simulink model "Failure_management_system"  (R2022b)
settings: Solver=VariableStepAuto  StartTime=0.0  StopTime=100  RelTol=1e-3
model workspace (MAT data in the model file):
  SnqAcq_FailMaxC_C = 2
  SnqAcq_WarnMaxC_C = 150
  SnrAcq_FailCDec_C = 0.2
  SnrAcq_FailCInc_C = 0.2
  SnrAcq_WarnCDec_C = 0.01
  SnrAcq_WarnCInc_C = 0.01
  SnrAcq_sdlDgo_DiagSrv_C = 0.1
  SnrAcq_sdlLow_SnrRead_C = 0.02
  SnrAcq_vMaxClampHys_C = 0.14
  SnrAcq_vMaxClamp_C = 14
  SnrAcq_vMaxLim_C = 16
  SnrAcq_vMinClampHys_C = 0.1
  SnrAcq_vMinClamp_C = 10
  SnrAcq_vMinLim_C = 6
undefined symbols (not defined in the file): sigbuilder_block
libraries: simulink x3
settings Model: NumberOfSteps=20  Creator=Mohamed Wahdan  LastModifiedBy=Mohamed Wahdan

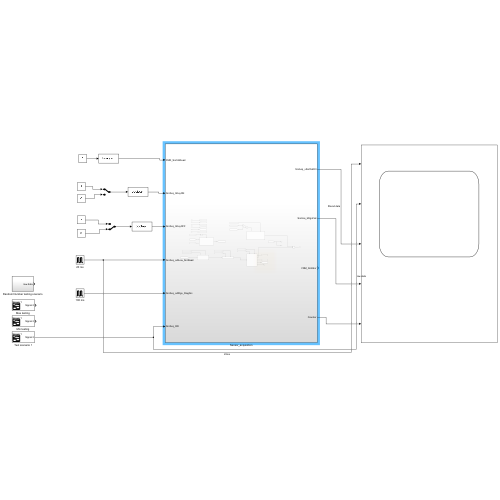
[thumbnail: Simulink's stored preview of the top-level diagram]
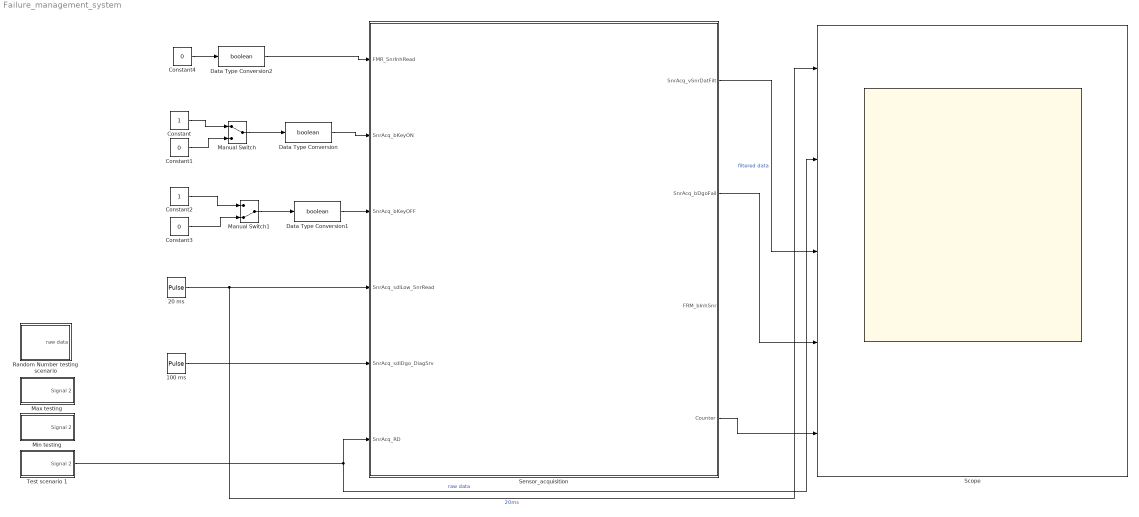
== system Failure_management_system ==
  100 ms : DiscretePulseGenerator  PulseType=Time based  Period=0.1  PulseWidth=50  SampleTime=SnrAcq_sdlDgo_DiagSrv_C
  20 ms : DiscretePulseGenerator  PulseType=Time based  Period=0.02  PulseWidth=50  SampleTime=SnrAcq_sdlLow_SnrRead_C
  Constant : Constant
  Constant1 : Constant  Value=0
  Constant2 : Constant
  Constant3 : Constant  Value=0
  Constant4 : Constant  Value=0
  Data Type Conversion : DataTypeConversion  OutDataTypeStr=boolean  SaturateOnIntegerOverflow=off  RndMeth=Floor
  Data Type Conversion1 : DataTypeConversion  OutDataTypeStr=boolean  SaturateOnIntegerOverflow=off  RndMeth=Floor
  Data Type Conversion2 : DataTypeConversion  OutDataTypeStr=boolean  SaturateOnIntegerOverflow=off  RndMeth=Floor
  Manual Switch : ManualSwitch
  Manual Switch1 : ManualSwitch  CurrentSetting=0
  "Max testing " : Subsystem  Tag=STV Subsys  LoadFcn=sigbuilder_block('load');  StartFcn=sigbuilder_block('start');  StopFcn=sigbuilder_block('stop');  ClipboardFcn=sigbuilder_block('clipboard');  mask(Sigbuilder block){tuvar=[0:10]}
      mask help: Simulink:masks:SigbuilderBlock_MD
      mask init:
      | if ~strcmp(get_param(bdroot(gcbh),'SimulationStatus'),'stopped') tuvar = sigbuilder_block('maskInit'); end
      settings: CopyFcn=sigbuilder_block('copy');  DeleteFcn=sigbuilder_block('delete');  ModelCloseFcn=sigbuilder_block('modelClose');  PreSaveFcn=sigbuilder_block('preSave');  PauseFcn=sigbuilder_block('pause');  ContinueFcn=sigbuilder_block('continue');  NameChangeFcn=sigbuilder_block('namechange');  OpenFcn=sigbuilder_block('open',[6 36 1428 675.75 ]);  CloseFcn=sigbuilder_block('close');
      mask Display: plot(0, 0, 100, 100,[2, 2, 32, 32, 2], [68, 8, 8, 68, 68],[32, 2], [38, 38], [32, 19, 2],[53, 60, 44], [32, 17, 17, 2],[16, 16, 31, 31]);txt = getActiveGroup(gcbh);text(2, 100, txt,'verticalAlignment', 'top');
  "Min testing " : Subsystem  Tag=STV Subsys  LoadFcn=sigbuilder_block('load');  StartFcn=sigbuilder_block('start');  StopFcn=sigbuilder_block('stop');  ClipboardFcn=sigbuilder_block('clipboard');  mask(Sigbuilder block){tuvar=[0:10]}
      mask help: Simulink:masks:SigbuilderBlock_MD
      mask init:
      | if ~strcmp(get_param(bdroot(gcbh),'SimulationStatus'),'stopped') tuvar = sigbuilder_block('maskInit'); end
      settings: CopyFcn=sigbuilder_block('copy');  DeleteFcn=sigbuilder_block('delete');  ModelCloseFcn=sigbuilder_block('modelClose');  PreSaveFcn=sigbuilder_block('preSave');  PauseFcn=sigbuilder_block('pause');  ContinueFcn=sigbuilder_block('continue');  NameChangeFcn=sigbuilder_block('namechange');  OpenFcn=sigbuilder_block('open',[6 36 1428 675.75 ]);  CloseFcn=sigbuilder_block('close');
      mask Display: plot(0, 0, 100, 100,[2, 2, 32, 32, 2], [68, 8, 8, 68, 68],[32, 2], [38, 38], [32, 19, 2],[53, 60, 44], [32, 17, 17, 2],[16, 16, 31, 31]);txt = getActiveGroup(gcbh);text(2, 100, txt,'verticalAlignment', 'top');
  Random Number testing scenario : Subsystem
  Scope : Scope  NumInputPorts=5
  Sensor_acquisition : Subsystem
  Test scenario 1 : Subsystem  Tag=STV Subsys  LoadFcn=sigbuilder_block('load');  StartFcn=sigbuilder_block('start');  StopFcn=sigbuilder_block('stop');  ClipboardFcn=sigbuilder_block('clipboard');  mask(Sigbuilder block){tuvar=[0:10]}
      mask help: Simulink:masks:SigbuilderBlock_MD
      mask init:
      | if ~strcmp(get_param(bdroot(gcbh),'SimulationStatus'),'stopped') tuvar = sigbuilder_block('maskInit'); end
      settings: CopyFcn=sigbuilder_block('copy');  DeleteFcn=sigbuilder_block('delete');  ModelCloseFcn=sigbuilder_block('modelClose');  PreSaveFcn=sigbuilder_block('preSave');  PauseFcn=sigbuilder_block('pause');  ContinueFcn=sigbuilder_block('continue');  NameChangeFcn=sigbuilder_block('namechange');  OpenFcn=sigbuilder_block('open',[6 36 1428 675.75 ]);  CloseFcn=sigbuilder_block('close');
      mask Display: plot(0, 0, 100, 100,[2, 2, 32, 32, 2], [68, 8, 8, 68, 68],[32, 2], [38, 38], [32, 19, 2],[53, 60, 44], [32, 17, 17, 2],[16, 16, 31, 31]);txt = getActiveGroup(gcbh);text(2, 100, txt,'verticalAlignment', 'top');
  wires:
  20 ms/1 -> Scope/1, Sensor_acquisition/4(SnrAcq_sdlLow_SnrRead)  "20ms"
  100 ms/1 -> Sensor_acquisition/5(SnrAcq_sdlDgo_DiagSrv)
  Constant1/1 -> Manual Switch/2
  Constant/1 -> Manual Switch/1
  Manual Switch/1 -> Data Type Conversion/1
  Data Type Conversion/1 -> Sensor_acquisition/2(SnrAcq_bKeyON)
  Manual Switch1/1 -> Data Type Conversion1/1
  Constant2/1 -> Manual Switch1/1
  Constant3/1 -> Manual Switch1/2
  Data Type Conversion1/1 -> Sensor_acquisition/3(SnrAcq_bKeyOFF)
  Constant4/1 -> Data Type Conversion2/1
  Data Type Conversion2/1 -> Sensor_acquisition/1(FMR_SnrInhRead)
  Sensor_acquisition/1(SnrAcq_vSnrDatFilt) -> Scope/3  "filtered data"
  Test scenario 1/1(Signal 2) -> Sensor_acquisition/6(SnrAcq_RD), Scope/2  "raw data"
  Sensor_acquisition/2(SnrAcq_bDgoFail) -> Scope/4
  Sensor_acquisition/4(Counter) -> Scope/5

== system Failure_management_system/Max testing  ==
  Demux : Demux  Tag=STV Demux  Outputs=1
      settings: DisplayOption=none
  FromWs : FromWorkspace  Tag=STV FromWs  VariableName=tuvar
      SigBuilderData=|
      | common.afterFinalStr = 'Extrapolate'
      | common.sampleTime = 0
      | dataSet.timeRange = [0 100]
      | dataSet.name = 'Group 1'
      | sbobj.Groups.Name = 'Group 1'
      | sbobj.Groups.Signals.Name = 'Signal 2'
      | sbobj.Groups.Signals.XData = [0 20 20 60 60 100]
      | sbobj.Groups.Signals.YData = [12 12 17 17 12 12]
      | sbobj.Groups.TimeRange = [0 100]
  Signal 2 : Outport  Tag=STV Outport
  wires:
  FromWs/1 -> Demux/1
  Demux/1 -> Signal 2/1

== system Failure_management_system/Min testing  ==
  Demux : Demux  Tag=STV Demux  Outputs=1
      settings: DisplayOption=none
  FromWs : FromWorkspace  Tag=STV FromWs  VariableName=tuvar
      SigBuilderData=|
      | common.afterFinalStr = 'Extrapolate'
      | common.sampleTime = 0
      | dataSet.timeRange = [0 100]
      | dataSet.name = 'Group 1'
      | sbobj.Groups.Name = 'Group 1'
      | sbobj.Groups.Signals.Name = 'Signal 2'
      | sbobj.Groups.Signals.XData = [0 20 20 60 60 100]
      | sbobj.Groups.Signals.YData = [12 12 5 5 12 12]
      | sbobj.Groups.TimeRange = [0 100]
  Signal 2 : Outport  Tag=STV Outport
  wires:
  Demux/1 -> Signal 2/1
  FromWs/1 -> Demux/1

== system Failure_management_system/Random Number testing scenario ==
  Add : Sum
  Random Number : RandomNumber  Mean=12  Variance=5  SampleTime=1
  Sine Wave : Sin  SampleTime=0.2
  raw data : Outport
  wires:
  Random Number/1 -> Add/2
  Add/1 -> raw data/1  "raw data"
  Sine Wave/1 -> Add/1

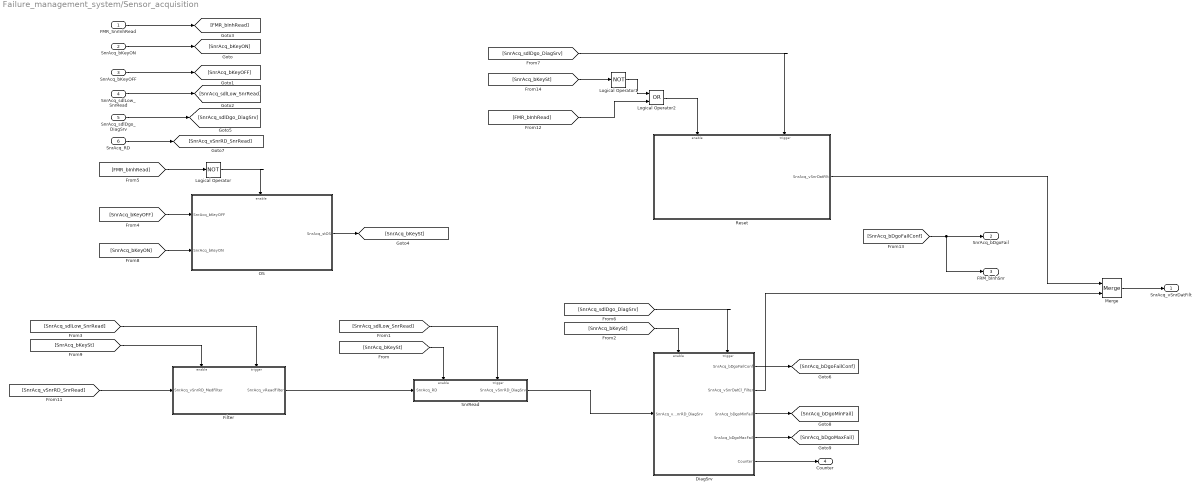
== system Failure_management_system/Sensor_acquisition ==
  FMR_SnrInhRead : Inport
  SnrAcq_bKeyON : Inport  Port=2
  SnrAcq_bKeyOFF : Inport  Port=3
  SnrAcq_sdlLow_SnrRead : Inport  Port=4
  SnrAcq_sdlDgo_DiagSrv : Inport  Port=5
  SnrAcq_RD : Inport  Port=6
  DiagSrv : Subsystem  TreatAsAtomicUnit=on
  Filter : Subsystem  TreatAsAtomicUnit=on
  Logical Operator : Logic  Operator=NOT  AllPortsSameDT=off  OutDataTypeStr=boolean
  Logical Operator1 : Logic  Operator=NOT  AllPortsSameDT=off  OutDataTypeStr=boolean
  Logical Operator2 : Logic  Operator=OR  AllPortsSameDT=off  OutDataTypeStr=boolean
  Merge : Merge
  OS : Subsystem  TreatAsAtomicUnit=on
  Reset : Subsystem  TreatAsAtomicUnit=on
  SnrRead : Subsystem  TreatAsAtomicUnit=on
  SnrAcq_vSnrDatFilt : Outport
  SnrAcq_bDgoFail : Outport  Port=2
  FRM_bInhSnr : Outport  Port=3
  Counter : Outport  Port=4
  wires:
  SnrAcq_bKeyON/1 -> [SnrAcq_bKeyON]
  SnrAcq_bKeyOFF/1 -> [SnrAcq_bKeyOFF]
  [SnrAcq_bKeySt] -> SnrRead/Enable
  SnrAcq_sdlLow_SnrRead/1 -> [SnrAcq_sdlLow_SnrRead]
  [SnrAcq_sdlLow_SnrRead] -> SnrRead/Trigger
  [SnrAcq_sdlLow_SnrRead] -> Filter/Trigger
  [SnrAcq_bKeySt] -> Filter/Enable
  FMR_SnrInhRead/1 -> [FMR_bInhRead]
  SnrAcq_sdlDgo_DiagSrv/1 -> [SnrAcq_sdlDgo_DiagSrv]
  [SnrAcq_bKeyOFF] -> OS/1(SnrAcq_bKeyOFF)
  [FMR_bInhRead] -> Logical Operator/1
  SnrAcq_RD/1 -> [SnrAcq_vSnrRD_SnrRead]
  [SnrAcq_bKeyON] -> OS/2(SnrAcq_bKeyON)
  Filter/1(SnrAcq_vReadFilter) -> SnrRead/1(SnrAcq_RD)
  [SnrAcq_vSnrRD_SnrRead] -> Filter/1(SnrAcq_vSnrRD_MedFilter)
  OS/1(SnrAcq_stOS) -> [SnrAcq_bKeySt]
  Logical Operator/1 -> OS/Enable
  DiagSrv/2(SnrAcq_vSnrDatCl_Filter) -> Merge/2
  DiagSrv/4(SnrAcq_bDgoMaxFail) -> [SnrAcq_bDgoMaxFail]
  DiagSrv/1(SnrAcq_bDgoFailConf) -> [SnrAcq_bDgoFailConf]
  Logical Operator2/1 -> Reset/Enable
  [SnrAcq_sdlDgo_DiagSrv] -> Reset/Trigger
  Reset/1(SnrAcq_vSnrDatFilt) -> Merge/1
  [SnrAcq_bKeySt] -> DiagSrv/Enable
  Merge/1 -> SnrAcq_vSnrDatFilt/1
  Logical Operator1/1 -> Logical Operator2/1
  [SnrAcq_bDgoFailConf] -> SnrAcq_bDgoFail/1, FRM_bInhSnr/1
  DiagSrv/3(SnrAcq_bDgoMinFail) -> [SnrAcq_bDgoMinFail]
  [FMR_bInhRead] -> Logical Operator2/2
  [SnrAcq_bKeySt] -> Logical Operator1/1
  [SnrAcq_sdlDgo_DiagSrv] -> DiagSrv/Trigger
  SnrRead/1(SnrAcq_vSnrRD_DiagSrv) -> DiagSrv/1(SnrAcq_vSnrRD_DiagSrv)
  DiagSrv/5(Counter) -> Counter/1

== system Failure_management_system/Test scenario 1 ==
  Demux : Demux  Tag=STV Demux  Outputs=1
      settings: DisplayOption=none
  FromWs : FromWorkspace  Tag=STV FromWs  VariableName=tuvar
      SigBuilderData=|
      | common.afterFinalStr = 'Extrapolate'
      | common.sampleTime = 0
      | dataSet.timeRange = [0 100]
      | dataSet.name = 'Group 1'
      | sbobj.Groups.Name = 'Group 1'
      | sbobj.Groups.Signals.Name = 'Signal 2'
      | sbobj.Groups.Signals.XData = [0 20 20 30 30 35 35 44.5 44.5 50 50 55 55 65 65 74.9 100]
      | sbobj.Groups.Signals.YData = [12 12 13.24 13.24 12 12 10 10 11 11 6 6 5 5 10 13.96 13.94]
      | sbobj.Groups.TimeRange = [0 100]
  Signal 2 : Outport  Tag=STV Outport
  wires:
  FromWs/1 -> Demux/1
  Demux/1 -> Signal 2/1

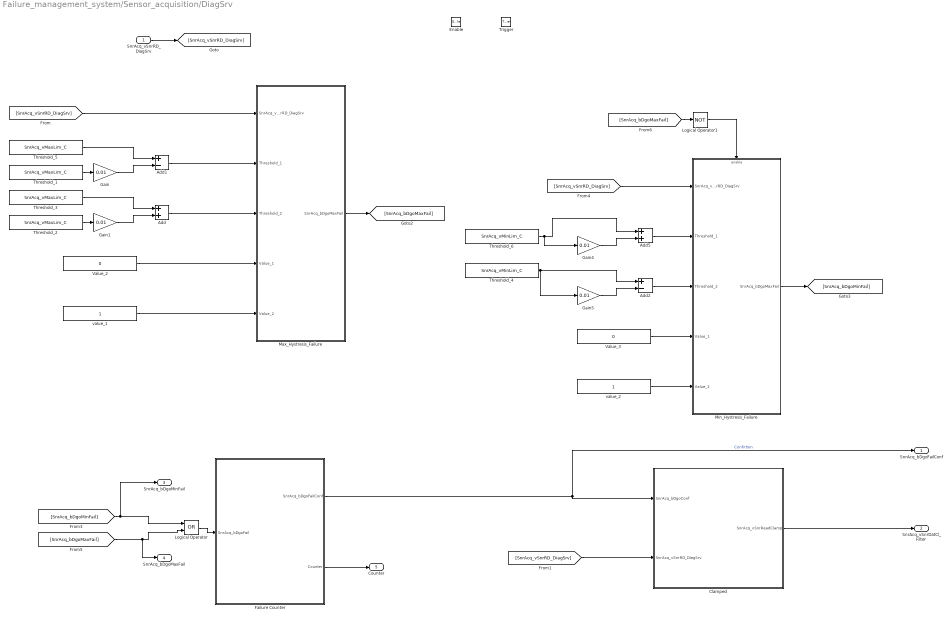
== system Failure_management_system/Sensor_acquisition/DiagSrv ==
  SnrAcq_vSnrRD_DiagSrv : Inport
  Enable : EnablePort
  Trigger : TriggerPort  VariantControl=(inherit)
  Add : Sum
  Add1 : Sum  Inputs=+-
  Add2 : Sum  Inputs=+-
  Add5 : Sum
  "Clamped " : Subsystem  TreatAsAtomicUnit=on
  Failure Counter : Subsystem
  Gain{,1,4..5} (4 alike) : Gain  Gain=0.01
  Logical Operator : Logic  Operator=OR  AllPortsSameDT=off  OutDataTypeStr=boolean
  Logical Operator1 : Logic  Operator=NOT  AllPortsSameDT=off  OutDataTypeStr=boolean
  Max_Hystresis_Failure : Subsystem
  Min_Hystresis_Failure : Subsystem
  Threshold_{1..3,5} (4 alike) : Constant  Value=SnrAcq_vMaxLim_C
  Threshold_4 : Constant  Value=SnrAcq_vMinLim_C
  Threshold_6 : Constant  Value=SnrAcq_vMinLim_C
  Value_2 : Constant  Value=0
  Value_3 : Constant  Value=0
  value_1 : Constant
  value_2 : Constant
  SnrAcq_bDgoFailConf : Outport
  SnrAcq_vSnrDatCl_Filter : Outport  Port=2
  SnrAcq_bDgoMinFail : Outport  Port=3
  SnrAcq_bDgoMaxFail : Outport  Port=4
  Counter : Outport  Port=5
  wires:
  value_1/1 -> Max_Hystresis_Failure/5(Value_2)
  Add/1 -> Max_Hystresis_Failure/3(Threshold_2)
  Add1/1 -> Max_Hystresis_Failure/2(Threshold_1)
  Value_2/1 -> Max_Hystresis_Failure/4(Value_1)
  [SnrAcq_vSnrRD_DiagSrv] -> Max_Hystresis_Failure/1(SnrAcq_vSnrRD_DiagSrv)
  SnrAcq_vSnrRD_DiagSrv/1 -> [SnrAcq_vSnrRD_DiagSrv]
  Gain/1 -> Add1/2
  Threshold_5/1 -> Add1/1
  Threshold_1/1 -> Gain/1
  Threshold_2/1 -> Gain1/1
  Threshold_3/1 -> Add/1
  Gain1/1 -> Add/2
  Logical Operator1/1 -> Min_Hystresis_Failure/Enable
  Add5/1 -> Min_Hystresis_Failure/2(Threshold_1)
  Min_Hystresis_Failure/1(" SnrAcq_bDgoMaxFail") -> [SnrAcq_bDgoMinFail]
  Gain4/1 -> Add5/2
  Add2/1 -> Min_Hystresis_Failure/3(Threshold_2)
  Threshold_4/1 -> Gain5/1, Add2/1
  Threshold_6/1 -> Add5/1, Gain4/1
  Gain5/1 -> Add2/2
  [SnrAcq_bDgoMaxFail] -> SnrAcq_bDgoMaxFail/1, Logical Operator/2
  [SnrAcq_bDgoMinFail] -> SnrAcq_bDgoMinFail/1, Logical Operator/1
  Max_Hystresis_Failure/1(" SnrAcq_bDgoMaxFail") -> [SnrAcq_bDgoMaxFail]
  [SnrAcq_bDgoMaxFail] -> Logical Operator1/1
  [SnrAcq_vSnrRD_DiagSrv] -> Min_Hystresis_Failure/1(SnrAcq_vSnrRD_DiagSrv)
  value_2/1 -> Min_Hystresis_Failure/5(Value_2)
  Value_3/1 -> Min_Hystresis_Failure/4(Value_1)
  Logical Operator/1 -> Failure Counter/1(SnrAcq_bDgoFail)
  Failure Counter/1(SnrAcq_bDgoFailConf) -> "Clamped "/1(SnrAcq_bDgoConf), SnrAcq_bDgoFailConf/1  "Confirtion"
  [SnrAcq_vSnrRD_DiagSrv] -> "Clamped "/2(SnrAcq_vSnrRD_DiagSrv)
  "Clamped "/1(SnrAcq_vSnrReadClamp) -> SnrAcq_vSnrDatCl_Filter/1
  Failure Counter/2(Counter) -> Counter/1

== system Failure_management_system/Sensor_acquisition/Filter ==
  SnrAcq_vSnrRD_MedFilter : Inport
  Enable : EnablePort
  Trigger : TriggerPort  TriggerType=either  VariantControl=(inherit)  PortDimensions=1
  Average : Subsystem
  Medfilter : Subsystem
  SnrAcq_vReadFilter : Outport  InitialOutput=12
  wires:
  SnrAcq_vSnrRD_MedFilter/1 -> Medfilter/1(SnrAcq_vSnrRD_MedFilter)
  Medfilter/1(SnrAcq_vMed_Avgfilter) -> Average/1(SnrAcq_vMed_Avgfilter)
  Average/1(SnrAcq_vReadFilter) -> SnrAcq_vReadFilter/1

== system Failure_management_system/Sensor_acquisition/OS ==
  SnrAcq_bKeyOFF : Inport
  SnrAcq_bKeyON : Inport  Port=2
  Enable : EnablePort
  Switch : Switch  Criteria=u2 ~= 0  SaturateOnIntegerOverflow=off  InputSameDT=off
  SnrAcq_stOS : Outport
  wires:
  SnrAcq_bKeyON/1 -> Switch/3
  SnrAcq_bKeyOFF/1 -> Switch/2, Switch/1
  Switch/1 -> SnrAcq_stOS/1

== system Failure_management_system/Sensor_acquisition/Reset ==
  Enable : EnablePort
  Trigger : TriggerPort  VariantControl=(inherit)
  Enabled Subsystem1 : Subsystem  TreatAsAtomicUnit=on
  SnrAcq_vSnrDatFilt : Outport
  wires:
  Enabled Subsystem1/1(SnrAcq_vSnrRst_SC) -> SnrAcq_vSnrDatFilt/1

== system Failure_management_system/Sensor_acquisition/SnrRead ==
  SnrAcq_RD : Inport
  Enable : EnablePort
  Trigger : TriggerPort  VariantControl=(inherit)
  Signal Conversion : SignalConversion  OverrideOpt=off
  SnrAcq_vSnrRD_DiagSrv : Outport  InitialOutput=12
  wires:
  SnrAcq_RD/1 -> Signal Conversion/1
  Signal Conversion/1 -> SnrAcq_vSnrRD_DiagSrv/1

== system Failure_management_system/Sensor_acquisition/DiagSrv/Clamped  ==
  SnrAcq_bDgoConf : Inport
  SnrAcq_vSnrRD_DiagSrv : Inport  Port=2
  Clamping Signal : Subsystem
  If : If  IfExpression=u1 ~= 0
  If Action Subsystem : Subsystem  TreatAsAtomicUnit=on
  Merge : Merge
  SnrAcq_vSnrReadClamp : Outport
  wires:
  Clamping Signal/1(SnrAcq_vSnrReadClamp) -> Merge/1
  SnrAcq_bDgoConf/1 -> If/1
  SnrAcq_vSnrRD_DiagSrv/1 -> Clamping Signal/1(SnrAcq_vSnrRD_DiagSrv), If Action Subsystem/1(SnrAcq_vSnrRD_DiagSrv)
  If/1 -> Clamping Signal/Action
  If/2 -> If Action Subsystem/Action
  If Action Subsystem/1(Out1) -> Merge/2
  Merge/1 -> SnrAcq_vSnrReadClamp/1

== system Failure_management_system/Sensor_acquisition/DiagSrv/Failure Counter ==
  SnrAcq_bDgoFail : Inport
  Confirmation Counter : Subsystem
  Constant1 : Constant
  Constant2 : Constant
  Data Type Conversion : DataTypeConversion  OutDataTypeStr=boolean  SaturateOnIntegerOverflow=off  RndMeth=Floor
  Data Type Conversion1 : DataTypeConversion  OutDataTypeStr=boolean  SaturateOnIntegerOverflow=off  RndMeth=Floor
  Logical Operator : Logic  Operator=NOT  AllPortsSameDT=off  OutDataTypeStr=boolean
  SnrAcq_bDgoFailConf : Outport
  Counter : Outport  Port=2
  wires:
  SnrAcq_bDgoFail/1 -> Data Type Conversion1/1, Data Type Conversion/1
  Constant2/1 -> Confirmation Counter/3(SnrAcq_FailCInc_C)
  Constant1/1 -> Confirmation Counter/4(SnrAcq_FailCDec_C)
  Data Type Conversion/1 -> Confirmation Counter/1(SnrAcq_EveEnaWC)
  Confirmation Counter/1(SnrAcq_bDgoConf) -> SnrAcq_bDgoFailConf/1
  Logical Operator/1 -> Confirmation Counter/2(Input)
  Data Type Conversion1/1 -> Logical Operator/1
  Confirmation Counter/2(Counter) -> Counter/1

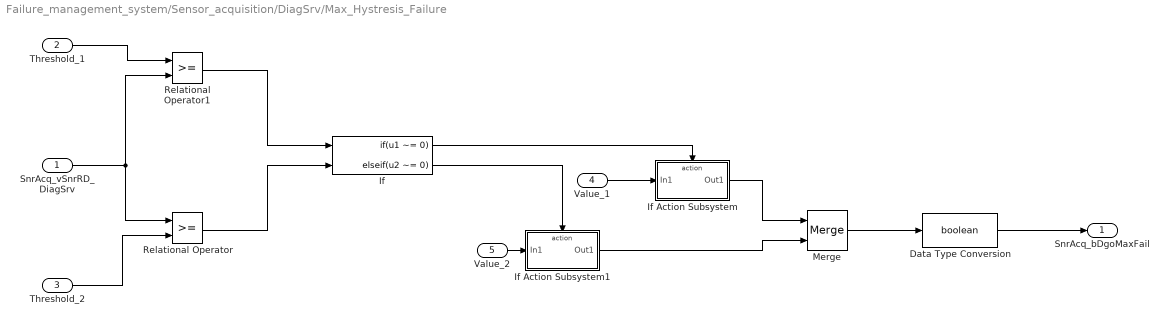
== system Failure_management_system/Sensor_acquisition/DiagSrv/Max_Hystresis_Failure ==
  SnrAcq_vSnrRD_DiagSrv : Inport
  Threshold_1 : Inport  Port=2
  Threshold_2 : Inport  Port=3
  Value_1 : Inport  Port=4
  Value_2 : Inport  Port=5
  Data Type Conversion : DataTypeConversion  OutDataTypeStr=boolean  SaturateOnIntegerOverflow=off  RndMeth=Floor
  If : If  NumInputs=2  IfExpression=u1 ~= 0  ElseIfExpressions=u2 ~= 0  ShowElse=off
  If Action Subsystem : Subsystem  TreatAsAtomicUnit=on
  If Action Subsystem1 : Subsystem  TreatAsAtomicUnit=on
  Merge : Merge
  Relational Operator : RelationalOperator  OutDataTypeStr=boolean  RndMeth=Simplest  InputSameDT=off
  Relational Operator1 : RelationalOperator  OutDataTypeStr=boolean  RndMeth=Simplest  InputSameDT=off
  " SnrAcq_bDgoMaxFail" : Outport
  wires:
  If/1 -> If Action Subsystem/Action
  Value_1/1 -> If Action Subsystem/1(In1)
  Value_2/1 -> If Action Subsystem1/1(In1)
  If/2 -> If Action Subsystem1/Action
  Merge/1 -> Data Type Conversion/1
  If Action Subsystem1/1(Out1) -> Merge/2
  If Action Subsystem/1(Out1) -> Merge/1
  Threshold_2/1 -> Relational Operator/2
  SnrAcq_vSnrRD_DiagSrv/1 -> Relational Operator1/2, Relational Operator/1
  Threshold_1/1 -> Relational Operator1/1
  Relational Operator/1 -> If/2
  Relational Operator1/1 -> If/1
  Data Type Conversion/1 -> " SnrAcq_bDgoMaxFail"/1

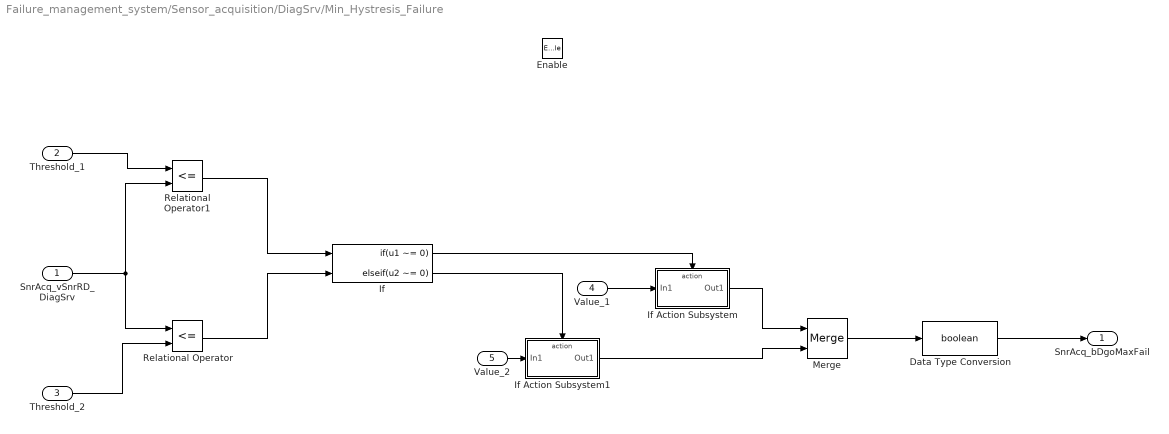
== system Failure_management_system/Sensor_acquisition/DiagSrv/Min_Hystresis_Failure ==
  SnrAcq_vSnrRD_DiagSrv : Inport
  Threshold_1 : Inport  Port=2
  Threshold_2 : Inport  Port=3
  Value_1 : Inport  Port=4
  Value_2 : Inport  Port=5
  Enable : EnablePort
  Data Type Conversion : DataTypeConversion  OutDataTypeStr=boolean  SaturateOnIntegerOverflow=off  RndMeth=Floor
  If : If  NumInputs=2  IfExpression=u1 ~= 0  ElseIfExpressions=u2 ~= 0  ShowElse=off
  If Action Subsystem : Subsystem  TreatAsAtomicUnit=on
  If Action Subsystem1 : Subsystem  TreatAsAtomicUnit=on
  Merge : Merge
  Relational Operator : RelationalOperator  Operator=<=  OutDataTypeStr=boolean  RndMeth=Simplest  InputSameDT=off
  Relational Operator1 : RelationalOperator  Operator=<=  OutDataTypeStr=boolean  RndMeth=Simplest  InputSameDT=off
  " SnrAcq_bDgoMaxFail" : Outport
  wires:
  Data Type Conversion/1 -> " SnrAcq_bDgoMaxFail"/1
  Relational Operator1/1 -> If/1
  Relational Operator/1 -> If/2
  Threshold_1/1 -> Relational Operator1/1
  SnrAcq_vSnrRD_DiagSrv/1 -> Relational Operator/1, Relational Operator1/2
  Threshold_2/1 -> Relational Operator/2
  If Action Subsystem/1(Out1) -> Merge/1
  If Action Subsystem1/1(Out1) -> Merge/2
  Merge/1 -> Data Type Conversion/1
  If/2 -> If Action Subsystem1/Action
  Value_2/1 -> If Action Subsystem1/1(In1)
  Value_1/1 -> If Action Subsystem/1(In1)
  If/1 -> If Action Subsystem/Action

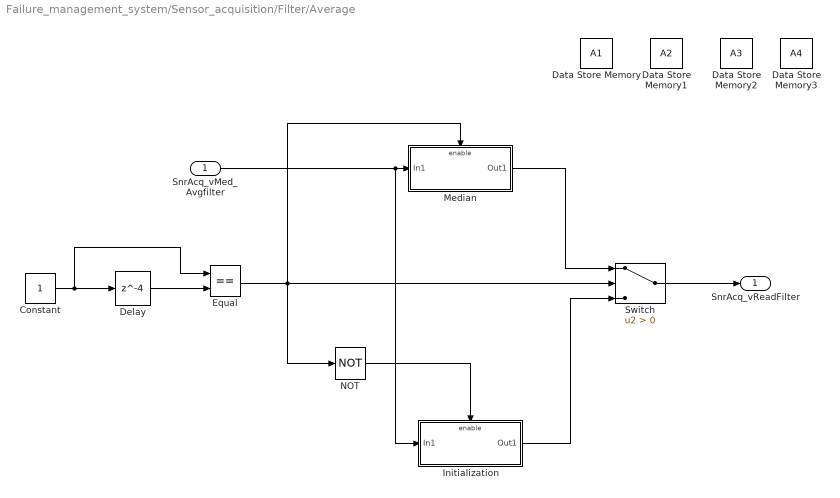
== system Failure_management_system/Sensor_acquisition/Filter/Average ==
  SnrAcq_vMed_Avgfilter : Inport
  Constant : Constant
  Data Store Memory : DataStoreMemory  DataStoreName=A1  ReadBeforeWriteMsg=warning  WriteAfterWriteMsg=warning  WriteAfterReadMsg=warning  ShowAdditionalParam=off
  Data Store Memory1 : DataStoreMemory  DataStoreName=A2  ReadBeforeWriteMsg=warning  WriteAfterWriteMsg=warning  WriteAfterReadMsg=warning  ShowAdditionalParam=off
  Data Store Memory2 : DataStoreMemory  DataStoreName=A3  ReadBeforeWriteMsg=warning  WriteAfterWriteMsg=warning  WriteAfterReadMsg=warning  ShowAdditionalParam=off
  Data Store Memory3 : DataStoreMemory  DataStoreName=A4  ReadBeforeWriteMsg=warning  WriteAfterWriteMsg=warning  WriteAfterReadMsg=warning  ShowAdditionalParam=off
  Delay : Delay  DelayLength=4
  Equal : RelationalOperator  Operator===  OutDataTypeStr=boolean  RndMeth=Simplest  InputSameDT=off
  Initialization : Subsystem
  Median : Subsystem
  NOT : Logic  Operator=NOT  IconShape=distinctive  AllPortsSameDT=off  OutDataTypeStr=boolean
  Switch : Switch  Criteria=u2 > Threshold  SaturateOnIntegerOverflow=off  InputSameDT=off
  SnrAcq_vReadFilter : Outport  VectorParamsAs1DForOutWhenUnconnected=off
  wires:
  Delay/1 -> Equal/2
  Constant/1 -> Equal/1, Delay/1
  NOT/1 -> Initialization/Enable
  SnrAcq_vMed_Avgfilter/1 -> Initialization/1(In1), Median/1(In1)
  Equal/1 -> Median/Enable, Switch/2, NOT/1
  Initialization/1(Out1) -> Switch/3
  Median/1(Out1) -> Switch/1
  Switch/1 -> SnrAcq_vReadFilter/1

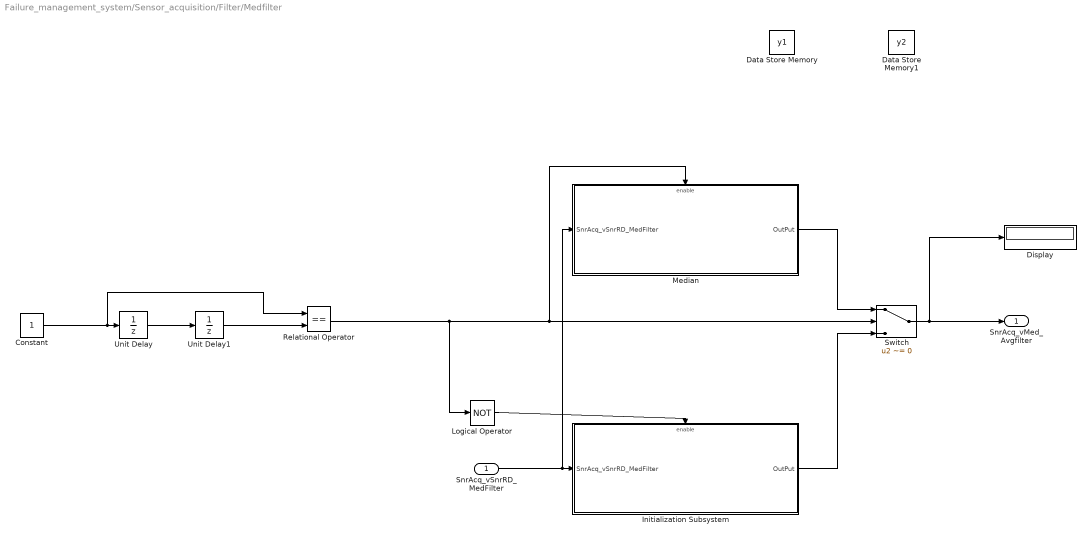
== system Failure_management_system/Sensor_acquisition/Filter/Medfilter ==
  SnrAcq_vSnrRD_MedFilter : Inport
  Constant : Constant
  Data Store Memory : DataStoreMemory  DataStoreName=y1  WriteAfterWriteMsg=warning  ShowAdditionalParam=off
  Data Store Memory1 : DataStoreMemory  DataStoreName=y2  WriteAfterWriteMsg=warning  ShowAdditionalParam=off
  Display : Display
  Initialization Subsystem : Subsystem  TreatAsAtomicUnit=on
  Logical Operator : Logic  Operator=NOT  AllPortsSameDT=off  OutDataTypeStr=boolean
  Median : Subsystem  TreatAsAtomicUnit=on
  Relational Operator : RelationalOperator  Operator===  OutDataTypeStr=boolean  RndMeth=Simplest  InputSameDT=off
  Switch : Switch  Criteria=u2 ~= 0  SaturateOnIntegerOverflow=off  InputSameDT=off
  Unit Delay : UnitDelay  SampleTime=-1  HasFrameUpgradeWarning=on
  Unit Delay1 : UnitDelay  SampleTime=-1  HasFrameUpgradeWarning=on
  SnrAcq_vMed_Avgfilter : Outport
  wires:
  Constant/1 -> Relational Operator/1, Unit Delay/1
  Unit Delay/1 -> Unit Delay1/1
  Unit Delay1/1 -> Relational Operator/2
  Relational Operator/1 -> Switch/2, Median/Enable, Logical Operator/1
  Logical Operator/1 -> Initialization Subsystem/Enable
  SnrAcq_vSnrRD_MedFilter/1 -> Median/1(SnrAcq_vSnrRD_MedFilter), Initialization Subsystem/1(SnrAcq_vSnrRD_MedFilter)
  Median/1(OutPut) -> Switch/1
  Initialization Subsystem/1(OutPut) -> Switch/3
  Switch/1 -> Display/1, SnrAcq_vMed_Avgfilter/1

== system Failure_management_system/Sensor_acquisition/Reset/Enabled Subsystem1 ==
  Constant : Constant  Value=12
  SnrAcq_vSnrRst_SC : Outport
  wires:
  Constant/1 -> SnrAcq_vSnrRst_SC/1

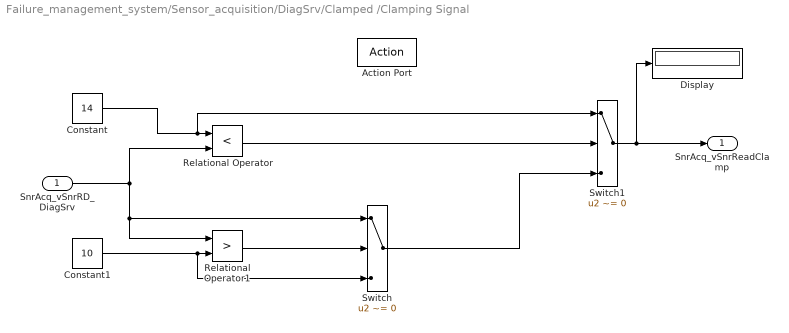
== system Failure_management_system/Sensor_acquisition/DiagSrv/Clamped /Clamping Signal ==
  SnrAcq_vSnrRD_DiagSrv : Inport
  Action Port : ActionPort  ActionPortLabel=if(u1 ~= 0)
  Constant : Constant  Value=14
  Constant1 : Constant  Value=10
  Display : Display
  Relational Operator : RelationalOperator  Operator=<  OutDataTypeStr=boolean  RndMeth=Simplest  InputSameDT=off
  Relational Operator1 : RelationalOperator  Operator=>  OutDataTypeStr=boolean  RndMeth=Simplest  InputSameDT=off
  Switch : Switch  Criteria=u2 ~= 0  SaturateOnIntegerOverflow=off  InputSameDT=off
  Switch1 : Switch  Criteria=u2 ~= 0  SaturateOnIntegerOverflow=off  InputSameDT=off
  SnrAcq_vSnrReadClamp : Outport
  wires:
  Constant/1 -> Switch1/1, Relational Operator/1
  SnrAcq_vSnrRD_DiagSrv/1 -> Switch/1, Relational Operator1/1, Relational Operator/2
  Constant1/1 -> Switch/3, Relational Operator1/2
  Relational Operator1/1 -> Switch/2
  Relational Operator/1 -> Switch1/2
  Switch/1 -> Switch1/3
  Switch1/1 -> Display/1, SnrAcq_vSnrReadClamp/1

== system Failure_management_system/Sensor_acquisition/DiagSrv/Clamped /If Action Subsystem ==
  SnrAcq_vSnrRD_DiagSrv : Inport
  Action Port : ActionPort  ActionPortLabel=else
  Out1 : Outport
  wires:
  SnrAcq_vSnrRD_DiagSrv/1 -> Out1/1

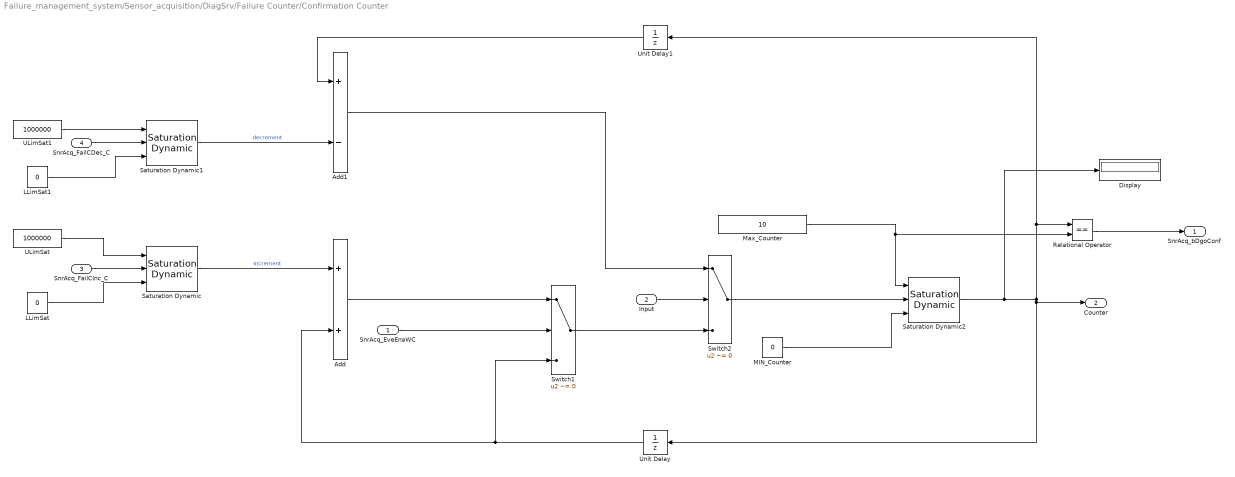
== system Failure_management_system/Sensor_acquisition/DiagSrv/Failure Counter/Confirmation Counter ==
  SnrAcq_EveEnaWC : Inport
  Input : Inport  Port=2
  SnrAcq_FailCInc_C : Inport  Port=3
  SnrAcq_FailCDec_C : Inport  Port=4
  Add : Sum
  Add1 : Sum  Inputs=+-
  Display : Display
  LLimSat : Constant  Value=0
  LLimSat1 : Constant  Value=0
  MIN_Counter : Constant  Value=0
  Max_Counter : Constant  Value=10
  Relational Operator : RelationalOperator  Operator===  OutDataTypeStr=boolean  RndMeth=Simplest  InputSameDT=off
  Saturation Dynamic : simulink/Discontinuities/Saturation Dynamic  OutMin=[]  OutMax=[]  OutDataTypeStr=Inherit: Same as second input  OutDataType=fixdt(1, 16)  OutScaling=2^-10  DoSatur=off
  Saturation Dynamic1 : simulink/Discontinuities/Saturation Dynamic  OutMin=[]  OutMax=[]  OutDataTypeStr=Inherit: Same as second input  OutDataType=fixdt(1, 16)  OutScaling=2^-10  DoSatur=off
  Saturation Dynamic2 : simulink/Discontinuities/Saturation Dynamic  OutMin=[]  OutMax=[]  OutDataTypeStr=Inherit: Same as second input  OutDataType=fixdt(1, 16)  OutScaling=2^-10  DoSatur=off
  Switch1 : Switch  Criteria=u2 ~= 0  SaturateOnIntegerOverflow=off  InputSameDT=off
  Switch2 : Switch  Criteria=u2 ~= 0  ZeroCross=off  SaturateOnIntegerOverflow=off  InputSameDT=off
  ULimSat : Constant  Value=1000000
  ULimSat1 : Constant  Value=1000000
  Unit Delay : UnitDelay  SampleTime=-1  HasFrameUpgradeWarning=on
  Unit Delay1 : UnitDelay  SampleTime=-1  HasFrameUpgradeWarning=on
  SnrAcq_bDgoConf : Outport
  Counter : Outport  Port=2
  wires:
  SnrAcq_FailCInc_C/1 -> Saturation Dynamic/2
  LLimSat/1 -> Saturation Dynamic/3
  ULimSat/1 -> Saturation Dynamic/1
  Saturation Dynamic/1 -> Add/1  "Increment"
  SnrAcq_EveEnaWC/1 -> Switch1/2
  Add/1 -> Switch1/1
  Unit Delay/1 -> Add/2, Switch1/3
  Switch1/1 -> Switch2/3
  Add1/1 -> Switch2/1
  Saturation Dynamic1/1 -> Add1/2  "decrement"
  ULimSat1/1 -> Saturation Dynamic1/1
  LLimSat1/1 -> Saturation Dynamic1/3
  SnrAcq_FailCDec_C/1 -> Saturation Dynamic1/2
  Unit Delay1/1 -> Add1/1
  Switch2/1 -> Saturation Dynamic2/2
  MIN_Counter/1 -> Saturation Dynamic2/3
  Max_Counter/1 -> Saturation Dynamic2/1, Relational Operator/2
  Saturation Dynamic2/1 -> Display/1, Counter/1, Unit Delay/1, Relational Operator/1, Unit Delay1/1
  Relational Operator/1 -> SnrAcq_bDgoConf/1
  Input/1 -> Switch2/2

== system Failure_management_system/Sensor_acquisition/DiagSrv/Max_Hystresis_Failure/If Action Subsystem ==
  In1 : Inport
  Action Port : ActionPort  ActionPortLabel=if(u1 ~= 0)
  Gain : Gain
  Out1 : Outport
  wires:
  In1/1 -> Gain/1
  Gain/1 -> Out1/1

== system Failure_management_system/Sensor_acquisition/DiagSrv/Max_Hystresis_Failure/If Action Subsystem1 ==
  In1 : Inport
  Action Port : ActionPort  ActionPortLabel=elseif(u2 ~= 0)
  Gain : Gain
  Out1 : Outport
  wires:
  In1/1 -> Gain/1
  Gain/1 -> Out1/1

== system Failure_management_system/Sensor_acquisition/DiagSrv/Min_Hystresis_Failure/If Action Subsystem ==
  In1 : Inport
  Action Port : ActionPort  ActionPortLabel=if(u1 ~= 0)
  Gain : Gain
  Out1 : Outport
  wires:
  Gain/1 -> Out1/1
  In1/1 -> Gain/1

== system Failure_management_system/Sensor_acquisition/DiagSrv/Min_Hystresis_Failure/If Action Subsystem1 ==
  In1 : Inport
  Action Port : ActionPort  ActionPortLabel=elseif(u2 ~= 0)
  Gain : Gain
  Out1 : Outport
  wires:
  Gain/1 -> Out1/1
  In1/1 -> Gain/1

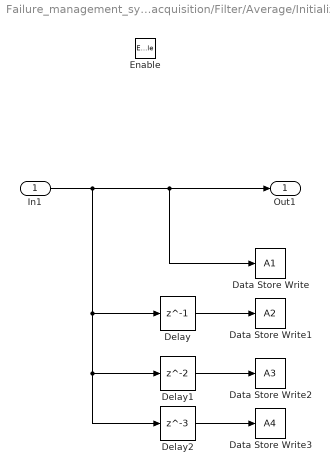
== system Failure_management_system/Sensor_acquisition/Filter/Average/Initialization ==
  In1 : Inport
  Enable : EnablePort
  Data Store Write : DataStoreWrite  DataStoreName=A1  IndexOptions=Index vector (dialog)  Indices=1  OutputSizes=1
  Data Store Write1 : DataStoreWrite  DataStoreName=A2  IndexOptions=Index vector (dialog)  Indices=1  OutputSizes=1
  Data Store Write2 : DataStoreWrite  DataStoreName=A3  IndexOptions=Index vector (dialog)  Indices=1  OutputSizes=1
  Data Store Write3 : DataStoreWrite  DataStoreName=A4  IndexOptions=Index vector (dialog)  Indices=1  OutputSizes=1
  Delay : Delay  DelayLength=1
  Delay1 : Delay
  Delay2 : Delay  DelayLength=3
  Out1 : Outport  VectorParamsAs1DForOutWhenUnconnected=off
  wires:
  In1/1 -> Delay2/1, Delay1/1, Delay/1, Out1/1, Data Store Write/1
  Delay/1 -> Data Store Write1/1
  Delay1/1 -> Data Store Write2/1
  Delay2/1 -> Data Store Write3/1

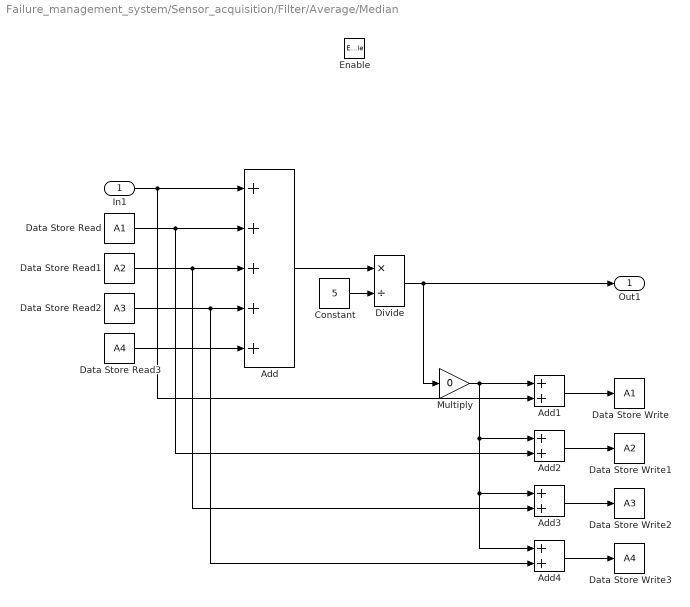
== system Failure_management_system/Sensor_acquisition/Filter/Average/Median ==
  In1 : Inport
  Enable : EnablePort
  Add : Sum  Inputs=5
  Add{1..4} (4 alike) : Sum
  Constant : Constant  Value=5
  Data Store Read : DataStoreRead  DataStoreName=A1  IndexOptions=Index vector (dialog)  Indices=1  OutputSizes=1
  Data Store Read1 : DataStoreRead  DataStoreName=A2  IndexOptions=Index vector (dialog)  Indices=1  OutputSizes=1
  Data Store Read2 : DataStoreRead  DataStoreName=A3  IndexOptions=Index vector (dialog)  Indices=1  OutputSizes=1
  Data Store Read3 : DataStoreRead  DataStoreName=A4  IndexOptions=Index vector (dialog)  Indices=1  OutputSizes=1
  Data Store Write : DataStoreWrite  DataStoreName=A1  IndexOptions=Index vector (dialog)  Indices=1  OutputSizes=1
  Data Store Write1 : DataStoreWrite  DataStoreName=A2  IndexOptions=Index vector (dialog)  Indices=1  OutputSizes=1
  Data Store Write2 : DataStoreWrite  DataStoreName=A3  IndexOptions=Index vector (dialog)  Indices=1  OutputSizes=1
  Data Store Write3 : DataStoreWrite  DataStoreName=A4  IndexOptions=Index vector (dialog)  Indices=1  OutputSizes=1
  Divide : Product  Inputs=*/
  Multiply : Gain  Gain=0
  Out1 : Outport  VectorParamsAs1DForOutWhenUnconnected=off
  wires:
  In1/1 -> Add/1, Add1/2
  Data Store Read/1 -> Add/2, Add2/2
  Data Store Read1/1 -> Add/3, Add3/2
  Data Store Read2/1 -> Add/4, Add4/2
  Data Store Read3/1 -> Add/5
  Add/1 -> Divide/1
  Constant/1 -> Divide/2
  Divide/1 -> Multiply/1, Out1/1
  Multiply/1 -> Add1/1, Add4/1, Add3/1, Add2/1
  Add1/1 -> Data Store Write/1
  Add2/1 -> Data Store Write1/1
  Add3/1 -> Data Store Write2/1
  Add4/1 -> Data Store Write3/1

== system Failure_management_system/Sensor_acquisition/Filter/Medfilter/Initialization Subsystem ==
  SnrAcq_vSnrRD_MedFilter : Inport
  Enable : EnablePort
  Data Store Write : DataStoreWrite  DataStoreName=y1  IndexOptions=Index vector (dialog)  Indices=1  OutputSizes=1
  Data Store Write1 : DataStoreWrite  DataStoreName=y2  IndexOptions=Index vector (dialog)  Indices=1  OutputSizes=1
  Unit Delay : UnitDelay  SampleTime=-1  HasFrameUpgradeWarning=on
  OutPut : Outport
  wires:
  SnrAcq_vSnrRD_MedFilter/1 -> Unit Delay/1, OutPut/1, Data Store Write/1
  Unit Delay/1 -> Data Store Write1/1

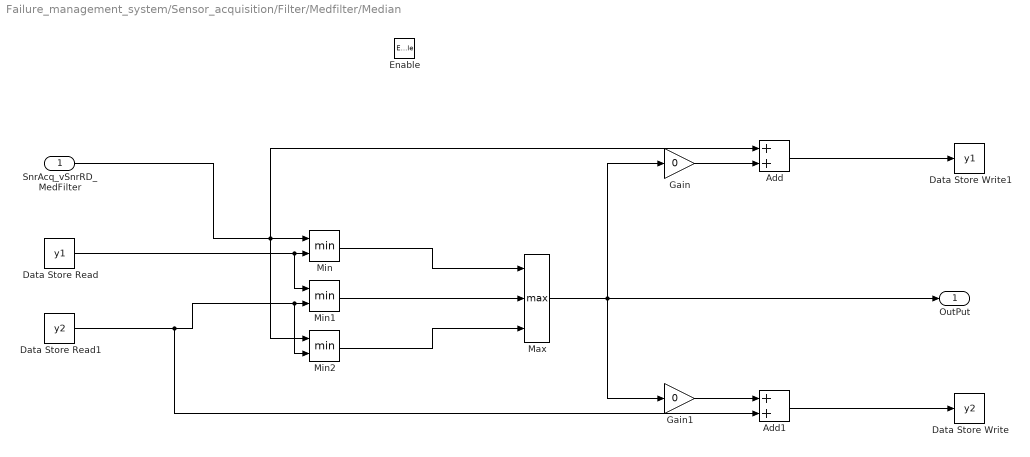
== system Failure_management_system/Sensor_acquisition/Filter/Medfilter/Median ==
  SnrAcq_vSnrRD_MedFilter : Inport
  Enable : EnablePort
  Add : Sum
  Add1 : Sum
  Data Store Read : DataStoreRead  DataStoreName=y1  IndexOptions=Index vector (dialog)  Indices=1  OutputSizes=1
  Data Store Read1 : DataStoreRead  DataStoreName=y2  IndexOptions=Index vector (dialog)  Indices=1  OutputSizes=1
  Data Store Write : DataStoreWrite  DataStoreName=y2  IndexOptions=Index vector (dialog)  Indices=1  OutputSizes=1
  Data Store Write1 : DataStoreWrite  DataStoreName=y1  IndexOptions=Index vector (dialog)  Indices=1  OutputSizes=1
  Gain : Gain  Gain=0
  Gain1 : Gain  Gain=0
  Max : MinMax  Function=max  Inputs=3
  Min : MinMax  Inputs=2
  Min1 : MinMax  Inputs=2
  Min2 : MinMax  Inputs=2
  OutPut : Outport
  wires:
  Min/1 -> Max/1
  Min1/1 -> Max/2
  Min2/1 -> Max/3
  SnrAcq_vSnrRD_MedFilter/1 -> Min/1, Min2/1, Add/1
  Data Store Read/1 -> Min1/1, Min/2
  Data Store Read1/1 -> Add1/2, Min2/2, Min1/2
  Add/1 -> Data Store Write1/1
  Gain/1 -> Add/2
  Max/1 -> Gain1/1, Gain/1, OutPut/1
  Gain1/1 -> Add1/1
  Add1/1 -> Data Store Write/1
